simulink model "closedLoop_Production"  (R2018a)
settings: Solver=VariableStepAuto  StartTime=0.0  StopTime=100  RelTol=1e-3
values from neighbouring files (symbols this model uses):
  A_Obs_est = A_est-L*C_est    [LQR_FeedBackRegulation.m]    (also in LQR_SetPoint_Regulation.m)
  B_Obs_est = [B_est-L*D_est L]    [LQR_FeedBackRegulation.m]    (also in LQR_SetPoint_Regulation.m)
  C_Obs_est = eye(4)    [LQR_FeedBackRegulation.m]    (also in LQR_SetPoint_Regulation.m)
  D_Obs_est = zeros(4,2)    [LQR_FeedBackRegulation.m]    (also in LQR_SetPoint_Regulation.m)
  k1 = (G_w0*W_np1^(2)*W_np2^(2))/(W_nz^(2))    [Esitmating_Plant_TF.m]    (also in LQR_FeedBackRegulation.m = K(1); LQR_SetPoint_Regulation.m = K(1); sineSweepOnVirtualPlant.m)
  k2 = K(2)    [LQR_FeedBackRegulation.m]    (also in LQR_SetPoint_Regulation.m)
  k3 = K(3)    [LQR_FeedBackRegulation.m]    (also in LQR_SetPoint_Regulation.m)
  k4 = K(4)    [LQR_FeedBackRegulation.m]    (also in LQR_SetPoint_Regulation.m)
  X0_Obs = [0 0 0 0]'    [LQR_FeedBackRegulation.m]    (also in LQR_SetPoint_Regulation.m)
settings Model: Creator=Dhruv  LastModifiedBy=ninadgaikwad
settings DataIOCC: SaveFinalState=on  SaveFormat=Structure  SaveState=on

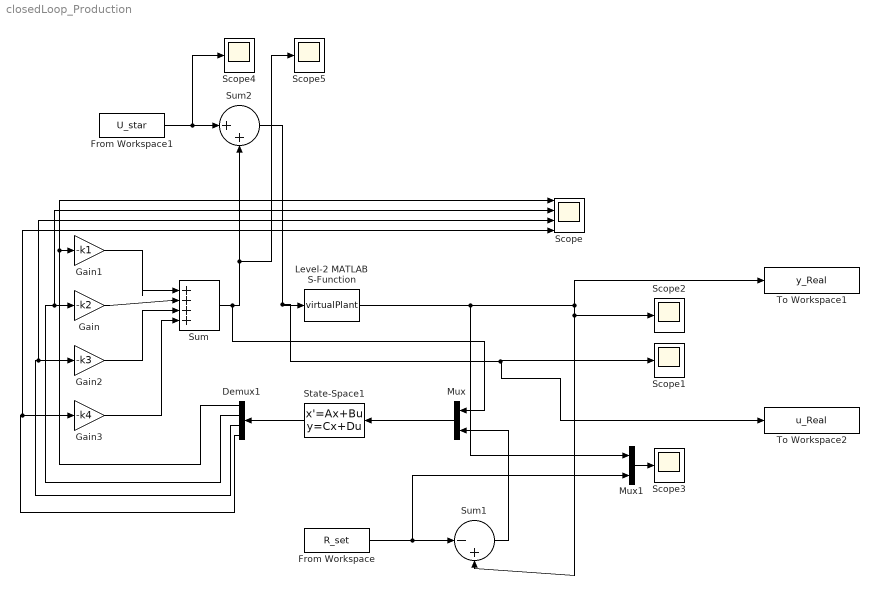
== system closedLoop_Production ==
  Demux1 : Demux
  From Workspace : FromWorkspace  VariableName=R_set  SampleTime=0
  From Workspace1 : FromWorkspace  VariableName=U_star  SampleTime=0
  Gain : Gain  Gain=-k2
  Gain1 : Gain  Gain=-k1
  Gain2 : Gain  Gain=-k3
  Gain3 : Gain  Gain=-k4
  Level-2 MATLAB S-Function : M-S-Function  FunctionName=virtualPlant
  Mux : Mux  Inputs=2
  Mux1 : Mux  Inputs=2
  Scope : Scope  NumInputPorts=4
  Scope{1..5} (5 alike) : Scope
  State-Space1 : StateSpace  A=A_Obs_est  B=B_Obs_est  C=C_Obs_est  D=D_Obs_est  InitialCondition=X0_Obs  ContinuousStateAttributes='Observer'
  Sum : Sum  Inputs=|++++
  Sum1 : Sum  Inputs=|-+
  Sum2 : Sum  Inputs=|++
  To Workspace1 : ToWorkspace  VariableName=y_Real  SampleTime=-1
  To Workspace2 : ToWorkspace  VariableName=u_Real  SampleTime=-1
  wires:
  Mux/1 -> State-Space1/1
  State-Space1/1 -> Demux1/1
  Gain1/1 -> Sum/1
  Gain/1 -> Sum/2
  Gain2/1 -> Sum/3
  Gain3/1 -> Sum/4
  Demux1/1 -> Scope/1, Gain1/1
  Demux1/2 -> Scope/2, Gain/1
  Demux1/4 -> Scope/4, Gain3/1
  Demux1/3 -> Scope/3, Gain2/1
  From Workspace/1 -> Mux1/2, Sum1/1
  Level-2 MATLAB S-Function/1 -> Mux1/1, Scope2/1, Sum1/2, To Workspace1/1
  Sum1/1 -> Mux/2
  From Workspace1/1 -> Scope4/1, Sum2/1
  Sum/1 -> Mux/1, Scope5/1, Sum2/2
  Sum2/1 -> Scope1/1, To Workspace2/1, Level-2 MATLAB S-Function/1
  Mux1/1 -> Scope3/1
